simulink model "velocity_time_distance"  (R2021a)
settings: Solver=VariableStepAuto  StartTime=0.0  StopTime=10.0  RelTol=1e-3
settings Model: Creator=MAC  LastModifiedBy=MAC

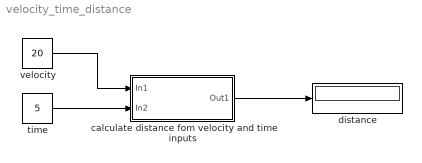
== system velocity_time_distance ==
  calculate distance fom velocity and time inputs : Subsystem
  distance : Display
  time : Constant  Value=5
  velocity : Constant  Value=20
  wires:
  velocity/1 -> calculate distance fom velocity and time inputs/1(In1)
  time/1 -> calculate distance fom velocity and time inputs/2(In2)
  calculate distance fom velocity and time inputs/1(Out1) -> distance/1

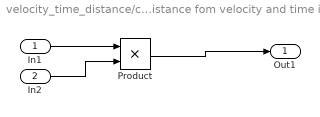
== system velocity_time_distance/calculate distance fom velocity and time inputs ==
  In1 : Inport
  In2 : Inport  Port=2
  Product : Product
  Out1 : Outport
  wires:
  In1/1 -> Product/1
  In2/1 -> Product/2
  Product/1 -> Out1/1
